simulink model "c2000_host_pfc"  (R2021b)
settings: Solver=VariableStepAuto  StartTime=0.0  StopTime=inf  RelTol=1e-3
libraries: instrumentseriallib x2, demo_controls x1
settings Model: Creator=The MathWorks, Inc.  LastModifiedBy=The MathWorks, Inc.
settings SolverCC: AlgebraicLoopSolver=TrustRegion
settings DebuggingCC: SymbolicDimsDataTypeCodeGenerationDiagnostic=none  SFMachineParentedDataDiag=warning

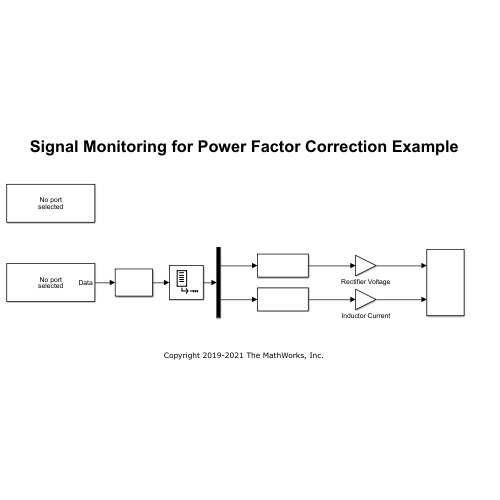
[thumbnail: Simulink's stored preview of the top-level diagram]
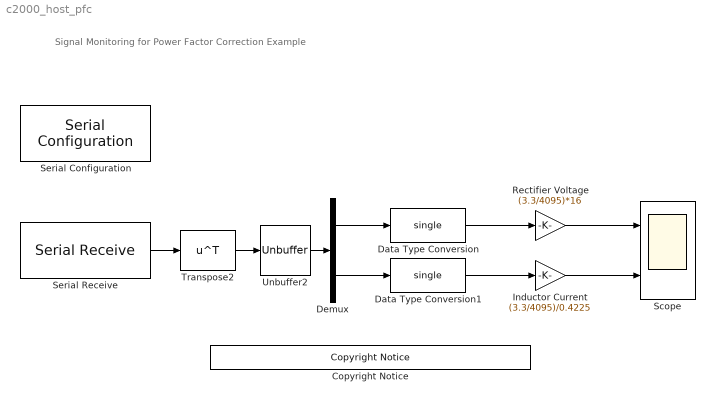
== system c2000_host_pfc ==
  note: Signal Monitoring for Power Factor Correction Example
  Copyright Notice : demo_controls/Copyright Notice  year=2019  prod=tic6000
      settings: SourceProductBaseCode=ME
  Data Type Conversion : DataTypeConversion  OutDataTypeStr=single
  Data Type Conversion1 : DataTypeConversion  OutDataTypeStr=single
  Demux : Demux  Outputs=2
  Inductor Current : Gain  Gain=(3.3/4095)/0.4225
  Rectifier Voltage : Gain  Gain=(3.3/4095)*16
  Scope : Scope  NumInputPorts=2
  Serial Configuration : instrumentseriallib/Serial Configuration  Priority=-200000  Port=<Select a port...>  ComPort=<Select a port...>  BaudRate=1500000  DataBits=8  Parity=none  StopBits=1  ByteOrder=little-endian  FlowControl=none  Timeout=10  SimulateUsing=Interpreted execution  BlockInModel=on
  Serial Receive : instrumentseriallib/Serial Receive  Port=<Select a port...>  ComPort=COM5  DataType=uint16  SaveDataType=uint8  ToggleHeader=on  Header="[ 83  83 ]"  ToggleTerminator=on  Terminator=Custom terminator  CustomTerminator="[ 69  69 ]"  ToggleDataSize=on  DataSize="[2  250]"  EnableBlockingMode=on  ActionDataUnavailable=Output last received value  ActionWhenDataUnavailable=Output last received value  CustomValue=0  SampleTime=0.05  SimulateUsing=Interpreted execution  BlockInModel=on
  Transpose2 : Math  Operator=transpose  SignedPower=on  SaturateOnIntegerOverflow=on
  Unbuffer2 : Unbuffer
  wires:
  Serial Receive/1 -> Transpose2/1
  Transpose2/1 -> Unbuffer2/1
  Unbuffer2/1 -> Demux/1
  Data Type Conversion1/1 -> Inductor Current/1
  Data Type Conversion/1 -> Rectifier Voltage/1
  Demux/1 -> Data Type Conversion/1
  Demux/2 -> Data Type Conversion1/1
  Rectifier Voltage/1 -> Scope/1
  Inductor Current/1 -> Scope/2
